simulink model "BLDC"  (R2020a)
settings: Solver=VariableStepAuto  StartTime=0.0  StopTime=10  RelTol=1e-3
libraries: nesl_utility x13, ee_lib x9, fl_lib x9
settings Model: Creator=sergio  LastModifiedBy=sergio

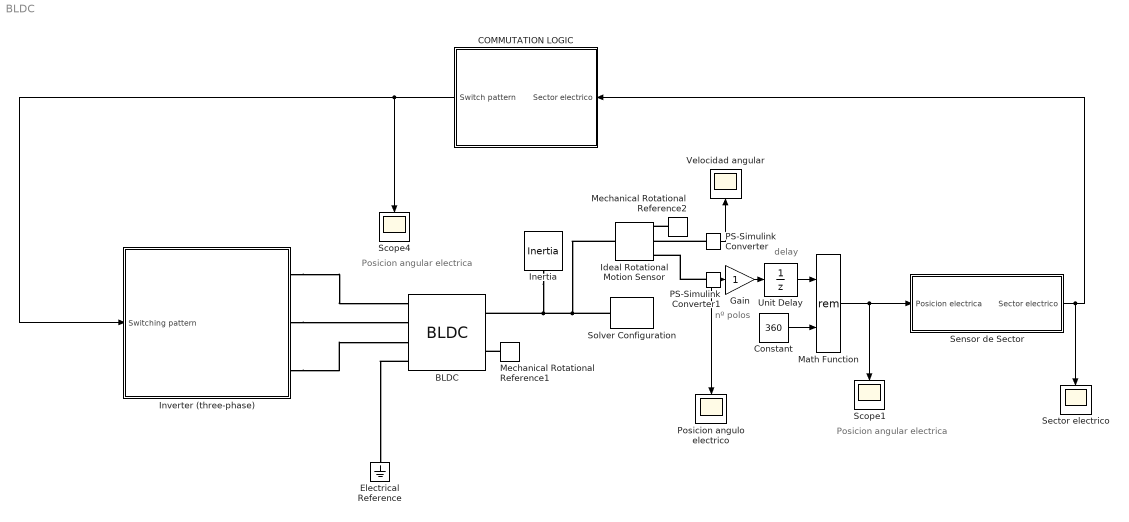
== system BLDC ==
  note: delay
  note: nº polos
  note: Posicion angular electrica
  note: Posicion angular electrica
  BLDC : ee_lib/Electromechanical/Permanent Magnet/BLDC  winding_type=ee.enum.statorconnection.wye  rotor_param=1  pm_flux_linkage=1 Wb  theta_constant=120 deg  emf_max=9.6 V  DphiDtheta_tab=[0, -.1528, -.1528, .1528, .1528, 0] Wb/rad  back_emf_tab=[0, -9.6, -9.6, 9.6, 9.6, 0] V  rotor_angle_tab=[0, 7.5, 22.5, 37.5, 52.5, 60] deg  w_meas=600 rpm  nPolePairs=1  stator_param=ee.enum.statorparam.LdLqL0  machine_param=ee.enum.dqparameterization.constant  Ld=8.5e-3 H  Lq=8.5e-3 H  idVec=[-200, 0, 200] A  iqVec=[-200, 0, 200] A  LdMatrix=0.00022 * ones(3, 3) H  LqMatrix=0.00022 * ones(3, 3) H  L0=0 H  Ls=0.0002 H  Lm=0 H  Ms=0.00002 H  Rs=0.04 Ohm  zero_sequence=ee.enum.park.zerosequence.include  J=0.01 kg*m^2  lam=0 N*m/(rad/s)  axes_param=2  i_d_specify=off  i_d_priority=None  i_d=0 A  i_d_nominal_specify=off  i_d_nominal_unit=A  i_d_nominal_value=1  i_q_specify=off  i_q_priority=None  i_q=0 A  i_q_nominal_specify=off  i_q_nominal_unit=A  i_q_nominal_value=1  torque_specify=off  torque_priority=None  torque=0 N*m  torque_nominal_specify=off  torque_nominal_unit=N*m  torque_nominal_value=1  angular_velocity_specify=off  angular_velocity_priority=High  angular_velocity=0 rpm  angular_velocity_nominal_specify=off  angular_velocity_nominal_unit=rpm  angular_velocity_nominal_value=1  angular_position_specify=off  angular_position_priority=High  angular_position=0 deg  angular_position_nominal_specify=off  angular_position_nominal_unit=deg  angular_position_nominal_value=1  loss_param=ee.enum.ironloss.none  losses_oc=[0, 0, 0] W  losses_sc=[0, 0, 0] W  f_losses=60 Hz  Isc_losses=95 A  Tmeas=298.15 K  alpha=3.93e-3 1/K  alpha_flux=-0.001 1/K  stator_thermal_mass=100 J/K  rotor_thermal_mass=200 J/K  Rm_percent_rotor=90  Rd_percent_rotor=30  temperatureA_specify=off  temperatureA_priority=High  temperatureA=25 degC  temperatureA_nominal_specify=off  temperatureA_nominal_unit=degC  temperatureA_nominal_value=1  temperatureB_specify=off  temperatureB_priority=High  temperatureB=25 degC  temperatureB_nominal_specify=off  temperatureB_nominal_unit=degC  temperatureB_nominal_value=1  temperatureC_specify=off  temperatureC_priority=High  temperatureC=25 degC  temperatureC_nominal_specify=off  temperatureC_nominal_unit=degC  temperatureC_nominal_value=1  temperatureR_specify=off  temperatureR_priority=High  temperatureR=25 degC  temperatureR_nominal_specify=off  temperatureR_nominal_unit=degC  temperatureR_nominal_value=1
      settings: SourceProductBaseCode=PS  InternalSimscapePortConfiguration="{\"Bottom\":[],\"Left\":[{\"id\":\"a\",\"label\":\"a\",\"type\":\"foundation.electrical.electrical\"},{\"id\":\"b\",\"label\":\"b\",\"type\":\"foundation.electrical.electrical\"},{\"id\":\"c\",\"label\":\"c\",\"type\":\"foundation.electrical.electrical\"},{\"id\":\"n\",\"label\":\"n\",\"type\":\"foundation.electrical.electrical\"}],\"Right\":[{\"id\":\"R\",\"label\":\"R\",\"type\":\"foundation.mechanical.rotational.rotational\"},{\"id\":\"C\",\"label\":\"C\",\"type\":\"foundation.mechanical.rotational.rotational\"}],\"Top\":[]}"
  COMMUTATION LOGIC : Subsystem
  Constant : Constant  Value=360
  Electrical Reference : fl_lib/Electrical/Electrical Elements/Electrical Reference
      settings: SourceProductBaseCode=MT,SS
  Gain : Gain
  Ideal Rotational Motion Sensor : fl_lib/Mechanical/Mechanical Sensors/Ideal Rotational Motion Sensor  wrap_angle=simscape.enum.onoff.on  offset=10 deg
  Inertia : fl_lib/Mechanical/Rotational Elements/Inertia  inertia=0.3 kg*m^2  w_specify=off  w_priority=High  w=0 rad/s  w_nominal_specify=off  w_nominal_unit=rad/s  w_nominal_value=1  t_specify=off  t_priority=None  t=0 N*m  t_nominal_specify=off  t_nominal_unit=N*m  t_nominal_value=1
  Inverter (three-phase) : Subsystem
  Math Function : Math  Operator=rem  SaturateOnIntegerOverflow=on
  Mechanical Rotational Reference1 : fl_lib/Mechanical/Rotational Elements/Mechanical Rotational Reference
  Mechanical Rotational Reference2 : fl_lib/Mechanical/Rotational Elements/Mechanical Rotational Reference
  PS-Simulink Converter : nesl_utility/PS-Simulink Converter  PhysicalDomain=network_engine_domain  SubClassName=ps_output  LeftPortType=input  RightPortType=output  PseudoPeriodic=off  Frequencies=[]  Unit=deg/s  AffineConversion=off
  PS-Simulink Converter1 : nesl_utility/PS-Simulink Converter  PhysicalDomain=network_engine_domain  SubClassName=ps_output  LeftPortType=input  RightPortType=output  PseudoPeriodic=off  Frequencies=[]  Unit=deg  AffineConversion=off
  Posicion angulo electrico : Scope
  Scope1 : Scope
  Scope4 : Scope
  Sector electrico : Scope
  Sensor de Sector : Subsystem
  Solver Configuration : nesl_utility/Solver Configuration  PhysicalDomain=network_engine_domain  SubClassName=solver  LeftPortType=input  RightPortType=generic  Tones=[]  Harmonics=[]  SimulateNoise=off  Profile=off  UseLocalSampling=off  EnableSwitchedLinearOptims=on  FrequencyDomain=off  UseCCode=off  RelTol=0.001  AbsTol=1e-06  MinStep=1e-09  ToWorkspace=off  RevertToSquareIcSolve=off  NumHomotopyIterations=100  PhasorMode=off  PhasorModeNumHarmonics=1  DoDC=off  ResidualTolerance=1e-09  UseLocalSolver=on  LocalSolverChoice=NE_BACKWARD_EULER_ADVANCER  LocalSolverSampleTime=0.001  DoFixedCost=on  MaxNonlinIter=3  MaxModeIter=2  LinearAlgebra=auto  EquationFormulation=NE_TIME_EF  DelaysMemoryBudget=1024  AutomaticFiltering=on  FilteringTimeConstant=0.001  PartitionStorageMethod=AS_NEEDED  PartitionMemoryBudget=1024  PartitionMethod=ROBUST
  Unit Delay : UnitDelay  SampleTime=-1  HasFrameUpgradeWarning=on
  Velocidad angular : Scope
  wires:
  PS-Simulink Converter/1 -> Velocidad angular/1
  Constant/1 -> Math Function/2
  Math Function/1 -> Scope1/1, Sensor de Sector/1(Posicion electrica)
  COMMUTATION LOGIC/1(Switch pattern) -> Inverter (three-phase)/1(Switching pattern), Scope4/1
  Sensor de Sector/1(Sector electrico) -> Sector electrico/1, COMMUTATION LOGIC/1(Sector electrico)
  Gain/1 -> Unit Delay/1
  Unit Delay/1 -> Math Function/1
  PS-Simulink Converter1/1 -> Posicion angulo electrico/1, Gain/1
  connections:
  BLDC/LConn4 -- Electrical Reference/LConn1
  Mechanical Rotational Reference1/LConn1 -- BLDC/RConn2
  Inverter (three-phase)/RConn1 -- BLDC/LConn1
  Inverter (three-phase)/RConn2 -- BLDC/LConn2
  Inverter (three-phase)/RConn3 -- BLDC/LConn3
  Solver Configuration/RConn1 -- Ideal Rotational Motion Sensor/LConn1 -- Inertia/LConn1 -- BLDC/RConn1
  Mechanical Rotational Reference2/LConn1 -- Ideal Rotational Motion Sensor/RConn1
  PS-Simulink Converter/LConn1 -- Ideal Rotational Motion Sensor/RConn2
  PS-Simulink Converter1/LConn1 -- Ideal Rotational Motion Sensor/RConn3

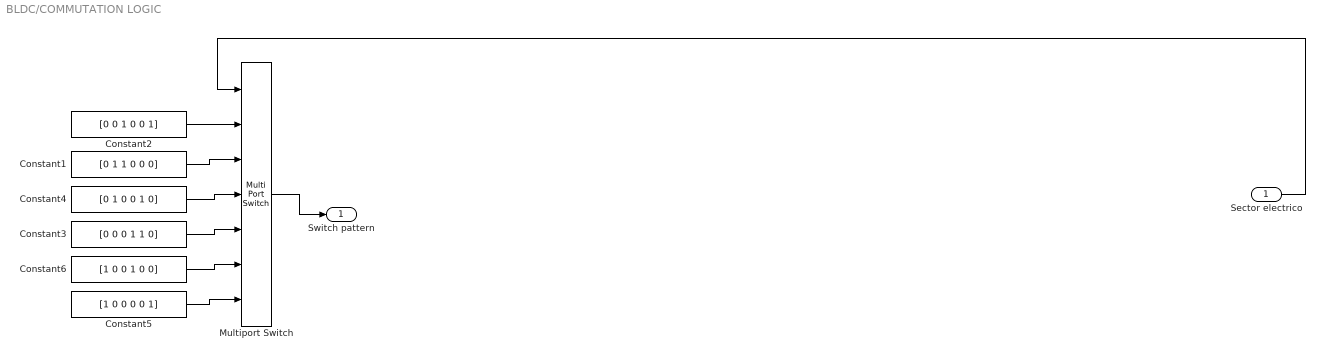
== system BLDC/COMMUTATION LOGIC ==
  Sector electrico : Inport
  Constant1 : Constant  Value=[0 1 1 0 0 0]
  Constant2 : Constant  Value=[0 0 1 0 0 1]
  Constant3 : Constant  Value=[0 0 0 1 1 0]
  Constant4 : Constant  Value=[0 1 0 0 1 0]
  Constant5 : Constant  Value=[1 0 0 0 0 1]
  Constant6 : Constant  Value=[1 0 0 1 0 0]
  Multiport Switch : MultiPortSwitch  Inputs=6  DiagnosticForDefault=Warning
  Switch pattern : Outport
  wires:
  Constant1/1 -> Multiport Switch/3
  Constant4/1 -> Multiport Switch/4
  Constant3/1 -> Multiport Switch/5
  Constant6/1 -> Multiport Switch/6
  Constant2/1 -> Multiport Switch/2
  Constant5/1 -> Multiport Switch/7
  Sector electrico/1 -> Multiport Switch/1
  Multiport Switch/1 -> Switch pattern/1

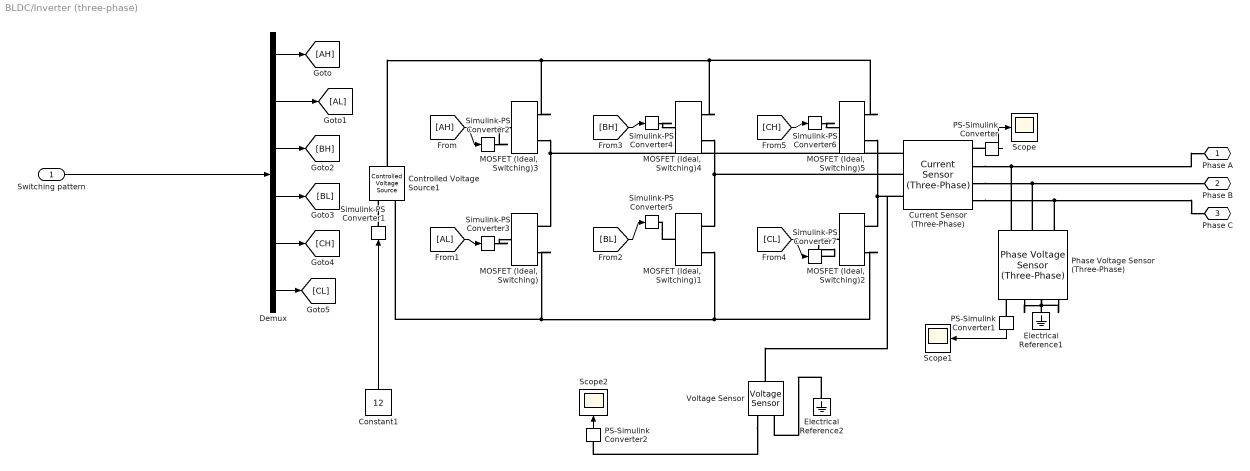
== system BLDC/Inverter (three-phase) ==
  Switching pattern : Inport
  Constant1 : Constant  Value=12
  Controlled Voltage Source1 : fl_lib/Electrical/Electrical Sources/Controlled Voltage Source
  Current Sensor (Three-Phase) : ee_lib/Sensors & Transducers/Current Sensor (Three-Phase)
      settings: InternalSimscapePortConfiguration="{\"Bottom\":[],\"Left\":[{\"id\":\"a1\",\"label\":\"a1\",\"type\":\"foundation.electrical.electrical\"},{\"id\":\"b1\",\"label\":\"b1\",\"type\":\"foundation.electrical.electrical\"},{\"id\":\"c1\",\"label\":\"c1\",\"type\":\"foundation.electrical.electrical\"}],\"Right\":[{\"id\":\"I_output\",\"label\":\"I\",\"type\":\"output\"},{\"id\":\"a2\",\"label\":\"a2\",\"type\":\"foundation.electrical.electrical\"},{\"id\":\"b2\",\"label\":\"b2\",\"type\":\"foundation.electrical.electrical\"},{\"id\":\"c2\",\"label\":\"c2\",\"type\":\"foundation.electrical.electrical\"}],\"Top\":[]}"
  Demux : Demux  Outputs=6
  Electrical Reference1 : fl_lib/Electrical/Electrical Elements/Electrical Reference
      settings: SourceProductBaseCode=MT,SS
  Electrical Reference2 : fl_lib/Electrical/Electrical Elements/Electrical Reference
      settings: SourceProductBaseCode=MT,SS
  MOSFET (Ideal, Switching){,1..5} (6 alike) : ee_lib/Semiconductors & Converters/MOSFET (Ideal, Switching)  Rds=0.01 Ohm  Goff=1e-6 1/Ohm  Vth=0.5 V  diode_param=2  diode_Vf=0.1 V  diode_Ron=0.001 Ohm  diode_Goff=1e-5 1/Ohm  diode_C=50e-9 F  diode_iRM=-235 A  diode_iF=300 A  diode_idot=-50 A/us  diode_trr_param=1  diode_trr_factor=3  diode_trr=15 us  diode_Qrr=1500 s*uA  thermal_loss_option=2  Voff=300 V  Tau=1e-4 s  Tj=[298.15, 398.15] K  Iout_scalar=600 A  Eon_scalar=22.86e-3 J  Eoff_scalar=17.14e-3 J  Von_scalar=2.7 V  Iout_data=[0, 10, 50, 100, 200, 400, 600] A  Eon_data=[0, .29, 1.43, 2.86, 5.71, 13.14, 22.86; 0, .57, 2.63, 5.14, 10.29, 20.57, 30.29] * 1e-3 J  Eoff_data=[0, .21, 1.07, 2.14, 4.29, 9.86, 17.14; 0, .43, 1.97, 3.86, 7.71, 15.43, 22.71] * 1e-3 J  Von_data=[0, 1.1, 1.3, 1.45, 1.75, 2.25, 2.7; 0, 1, 1.15, 1.35, 1.7, 2.35, 3] V
  PS-Simulink Converter : nesl_utility/PS-Simulink Converter  PhysicalDomain=network_engine_domain  SubClassName=ps_output  LeftPortType=input  RightPortType=output  PseudoPeriodic=off  Frequencies=[]  Unit=inherit  AffineConversion=off
  PS-Simulink Converter1 : nesl_utility/PS-Simulink Converter  PhysicalDomain=network_engine_domain  SubClassName=ps_output  LeftPortType=input  RightPortType=output  PseudoPeriodic=off  Frequencies=[]  Unit=inherit  AffineConversion=off
  PS-Simulink Converter2 : nesl_utility/PS-Simulink Converter  PhysicalDomain=network_engine_domain  SubClassName=ps_output  LeftPortType=input  RightPortType=output  PseudoPeriodic=off  Frequencies=[]  Unit=inherit  AffineConversion=off
  Phase Voltage Sensor (Three-Phase) : ee_lib/Sensors & Transducers/Phase Voltage Sensor (Three-Phase)
      settings: SourceProductBaseCode=PS  InternalSimscapePortConfiguration="{\"Bottom\":[],\"Left\":[{\"id\":\"a1\",\"label\":\"a1\",\"type\":\"foundation.electrical.electrical\"},{\"id\":\"b1\",\"label\":\"b1\",\"type\":\"foundation.electrical.electrical\"},{\"id\":\"c1\",\"label\":\"c1\",\"type\":\"foundation.electrical.electrical\"}],\"Right\":[{\"id\":\"V_output\",\"label\":\"V\",\"type\":\"output\"},{\"id\":\"a2\",\"label\":\"a2\",\"type\":\"foundation.electrical.electrical\"},{\"id\":\"b2\",\"label\":\"b2\",\"type\":\"foundation.electrical.electrical\"},{\"id\":\"c2\",\"label\":\"c2\",\"type\":\"foundation.electrical.electrical\"}],\"Top\":[]}"
  Scope : Scope
  Scope1 : Scope
  Scope2 : Scope
  Simulink-PS Converter1 : nesl_utility/Simulink-PS Converter  PhysicalDomain=network_engine_domain  SubClassName=ps_input  LeftPortType=input  RightPortType=output  PseudoPeriodic=off  Frequencies=[]  NoiseDistribution=none  NoiseParameters=[]  Unit=V  AffineConversion=off  FilteringAndDerivatives=provide  SimscapeFilterOrder=1  InputFilterTimeConstant=0.001  UdotUserProvided=0
  Simulink-PS Converter2 : nesl_utility/Simulink-PS Converter  PhysicalDomain=network_engine_domain  SubClassName=ps_input  LeftPortType=input  RightPortType=output  PseudoPeriodic=off  Frequencies=[]  NoiseDistribution=none  NoiseParameters=[]  Unit=V  AffineConversion=off  FilteringAndDerivatives=provide  SimscapeFilterOrder=1  InputFilterTimeConstant=0.001  UdotUserProvided=0
  Simulink-PS Converter{3..7} (5 alike) : nesl_utility/Simulink-PS Converter  PhysicalDomain=network_engine_domain  SubClassName=ps_input  LeftPortType=input  RightPortType=output  PseudoPeriodic=off  Frequencies=[]  NoiseDistribution=none  NoiseParameters=[]  Unit=1  AffineConversion=off  FilteringAndDerivatives=provide  SimscapeFilterOrder=1  InputFilterTimeConstant=0.001  UdotUserProvided=0
  Voltage Sensor : fl_lib/Electrical/Electrical Sensors/Voltage Sensor
  Phase A : PMIOPort  Side=Right
  Phase B : PMIOPort  Port=2  Side=Right
  Phase C : PMIOPort  Port=3  Side=Right
  wires:
  [AL] -> Simulink-PS Converter3/1
  PS-Simulink Converter/1 -> Scope/1
  [CL] -> Simulink-PS Converter7/1
  PS-Simulink Converter1/1 -> Scope1/1
  Demux/2 -> [AL]
  [BL] -> Simulink-PS Converter5/1
  Demux/5 -> [CH]
  [AH] -> Simulink-PS Converter2/1
  Demux/1 -> [AH]
  Switching pattern/1 -> Demux/1
  Demux/4 -> [BL]
  [CH] -> Simulink-PS Converter6/1
  Constant1/1 -> Simulink-PS Converter1/1
  [BH] -> Simulink-PS Converter4/1
  Demux/6 -> [CL]
  Demux/3 -> [BH]
  PS-Simulink Converter2/1 -> Scope2/1
  connections:
  Current Sensor (Three-Phase)/RConn4 -- Phase Voltage Sensor (Three-Phase)/LConn3 -- Phase C/RConn1
  Electrical Reference1/LConn1 -- Phase Voltage Sensor (Three-Phase)/RConn2 -- Phase Voltage Sensor (Three-Phase)/RConn3 -- Phase Voltage Sensor (Three-Phase)/RConn4
  "MOSFET (Ideal, Switching)1"/LConn1 -- Simulink-PS Converter5/RConn1
  "MOSFET (Ideal, Switching)3"/RConn1 -- Controlled Voltage Source1/LConn1 -- "MOSFET (Ideal, Switching)5"/RConn1 -- "MOSFET (Ideal, Switching)4"/RConn1
  Current Sensor (Three-Phase)/RConn2 -- Phase A/RConn1 -- Phase Voltage Sensor (Three-Phase)/LConn1
  "MOSFET (Ideal, Switching)4"/RConn2 -- Current Sensor (Three-Phase)/LConn2 -- "MOSFET (Ideal, Switching)1"/RConn1
  "MOSFET (Ideal, Switching)2"/LConn1 -- Simulink-PS Converter7/RConn1
  "MOSFET (Ideal, Switching)"/RConn2 -- Controlled Voltage Source1/RConn2 -- "MOSFET (Ideal, Switching)2"/RConn2 -- "MOSFET (Ideal, Switching)1"/RConn2
  Simulink-PS Converter1/RConn1 -- Controlled Voltage Source1/RConn1
  Current Sensor (Three-Phase)/RConn3 -- Phase B/RConn1 -- Phase Voltage Sensor (Three-Phase)/LConn2
  PS-Simulink Converter1/LConn1 -- Phase Voltage Sensor (Three-Phase)/RConn1
  "MOSFET (Ideal, Switching)3"/RConn2 -- Current Sensor (Three-Phase)/LConn1 -- "MOSFET (Ideal, Switching)"/RConn1
  PS-Simulink Converter/LConn1 -- Current Sensor (Three-Phase)/RConn1
  "MOSFET (Ideal, Switching)5"/RConn2 -- Voltage Sensor/LConn1 -- Current Sensor (Three-Phase)/LConn3 -- "MOSFET (Ideal, Switching)2"/RConn1
  Voltage Sensor/RConn1 -- PS-Simulink Converter2/LConn1
  Electrical Reference2/LConn1 -- Voltage Sensor/RConn2
  Simulink-PS Converter2/RConn1 -- "MOSFET (Ideal, Switching)3"/LConn1
  Simulink-PS Converter6/RConn1 -- "MOSFET (Ideal, Switching)5"/LConn1
  Simulink-PS Converter4/RConn1 -- "MOSFET (Ideal, Switching)4"/LConn1
  Simulink-PS Converter3/RConn1 -- "MOSFET (Ideal, Switching)"/LConn1

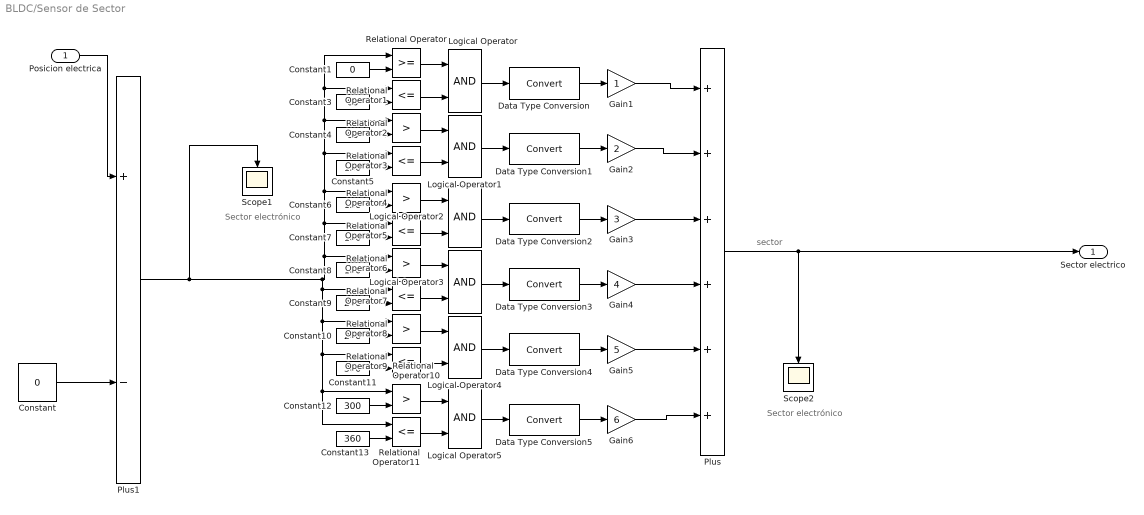
== system BLDC/Sensor de Sector ==
  note: sector
  note: Sector electrónico
  note: Sector electrónico
  Posicion electrica : Inport
  Constant : Constant  Value=0  VectorParams1D=off  SampleTime=-1
  Constant1 : Constant  Value=0
  Constant10 : Constant  Value=240
  Constant11 : Constant  Value=300
  Constant12 : Constant  Value=300
  Constant13 : Constant  Value=360
  Constant3 : Constant  Value=60
  Constant4 : Constant  Value=60
  Constant5 : Constant  Value=120
  Constant6 : Constant  Value=120
  Constant7 : Constant  Value=180
  Constant8 : Constant  Value=180
  Constant9 : Constant  Value=240
  Data Type Conversion{,1..5} (6 alike) : DataTypeConversion
  Gain1 : Gain
  Gain2 : Gain  Gain=2
  Gain3 : Gain  Gain=3
  Gain4 : Gain  Gain=4
  Gain5 : Gain  Gain=5
  Gain6 : Gain  Gain=6
  Logical Operator{,1..5} (6 alike) : Logic  AllPortsSameDT=off  OutDataTypeStr=boolean
  Plus : Sum  Inputs=++++++
  Plus1 : Sum  Inputs=+-
  Relational Operator : RelationalOperator  OutDataTypeStr=boolean  RndMeth=Simplest
  Relational Operator{1,3,5,7,9,11} (6 alike) : RelationalOperator  Operator=<=  OutDataTypeStr=boolean  RndMeth=Simplest
  Relational Operator{2,4,6,8,10} (5 alike) : RelationalOperator  Operator=>  OutDataTypeStr=boolean  RndMeth=Simplest
  Scope1 : Scope
  Scope2 : Scope
  Sector electrico : Outport
  wires:
  Logical Operator2/1 -> Data Type Conversion2/1
  Logical Operator/1 -> Data Type Conversion/1
  Relational Operator4/1 -> Logical Operator2/1
  Constant6/1 -> Relational Operator4/2
  Constant4/1 -> Relational Operator2/2
  Relational Operator5/1 -> Logical Operator2/2
  Data Type Conversion2/1 -> Gain3/1
  Gain5/1 -> Plus/5
  Constant12/1 -> Relational Operator10/2
  Constant8/1 -> Relational Operator6/2
  Plus/1 -> Sector electrico/1, Scope2/1
  Constant7/1 -> Relational Operator5/2
  Relational Operator/1 -> Logical Operator/1
  Relational Operator8/1 -> Logical Operator4/1
  Relational Operator2/1 -> Logical Operator1/1
  Relational Operator10/1 -> Logical Operator5/1
  Relational Operator7/1 -> Logical Operator3/2
  Gain6/1 -> Plus/6
  Relational Operator1/1 -> Logical Operator/2
  Constant10/1 -> Relational Operator8/2
  Data Type Conversion/1 -> Gain1/1
  Gain2/1 -> Plus/2
  Constant3/1 -> Relational Operator1/2
  Constant5/1 -> Relational Operator3/2
  Logical Operator3/1 -> Data Type Conversion3/1
  Relational Operator3/1 -> Logical Operator1/2
  Constant11/1 -> Relational Operator9/2
  Relational Operator11/1 -> Logical Operator5/2
  Data Type Conversion1/1 -> Gain2/1
  Logical Operator1/1 -> Data Type Conversion1/1
  Logical Operator5/1 -> Data Type Conversion5/1
  Constant1/1 -> Relational Operator/2
  Gain4/1 -> Plus/4
  Gain1/1 -> Plus/1
  Relational Operator6/1 -> Logical Operator3/1
  Logical Operator4/1 -> Data Type Conversion4/1
  Constant13/1 -> Relational Operator11/2
  Data Type Conversion4/1 -> Gain5/1
  Relational Operator9/1 -> Logical Operator4/2
  Data Type Conversion3/1 -> Gain4/1
  Gain3/1 -> Plus/3
  Constant9/1 -> Relational Operator7/2
  Data Type Conversion5/1 -> Gain6/1
  Posicion electrica/1 -> Plus1/1
  Plus1/1 -> Scope1/1, Relational Operator7/1, Relational Operator8/1, Relational Operator9/1, Relational Operator10/1, Relational Operator11/1, Relational Operator6/1, Relational Operator4/1, Relational Operator3/1, Relational Operator/1, Relational Operator1/1, Relational Operator2/1, Relational Operator5/1
  Constant/1 -> Plus1/2
